simulink model "TruckBenchmark"  (R2023a)
settings: Solver=FixedStepAuto  StartTime=0.0  StopTime=sim_time  FixedStep=control.Ts  MaxStep=1  RelTol=1e-3  EnableMultiTasking=on
StartFcn:
  | tic
StopFcn:
  | simt=toc;
  | fprintf('Simulation time %.3f s\n',simt)
  | TruckBenchmark_Evaluation
values from neighbouring files (symbols this model uses):
  attack_duration = input('Enter the duration of each attack: ')    [RunMe.m]
  attack_freq = input('Enter the desired frequency of attack: ')    [RunMe.m]
  attack_time = input('Enter the time for attack: ')    [RunMe.m]
  attack_type = input('Select the type of Attack (1= Fuzzy, 2=spoofing, 3=Plateau, 4=Replay Attack, 5 = GAttack, 6= C-GAttack, 7= No Attack, 8 = Denial of Service):')    [RunMe.m]
  can_sample_time = 0.001    [runSim.m]
  clutch_pos = TruckBenchmark_Result.find('clutch_pos').Values    [TruckBenchmark_Evaluation.m]
  control =     [TruckBenchmark_Control.mat]
  cruise_profile = input('Select Cruise Profile (Step decrease = 1, Constant 80kph = 2): ')    [RunMe.m]
  curr_gear = TruckBenchmark_Result.find('curr_gear').Values    [TruckBenchmark_Evaluation.m]
  DoS = 0    [RunMe.m]
  gattack_data = interp1(original_time, data, desired_time, 'linear')    [RunMe.m]
  gattack_time = desired_time    [RunMe.m]
  k_slope = TruckBenchmark_Result.find('k_slope').Values    [TruckBenchmark_Evaluation.m]
  lambda = TruckBenchmark_Result.find('lambda').Values    [TruckBenchmark_Evaluation.m]
  model =     [TruckBenchmark_Data.mat]
  n_engine = TruckBenchmark_Result.find('n_engine').Values    [TruckBenchmark_Evaluation.m]
  road = scenario.road    [runSim.m]
  scenario =     [Sodertalje_Norrkoping_Scenario.mat]
  sim_time = input('Enter the total simulation time: ')    [RunMe.m]
  spoofed_value = input('Set the spoofing value:')    [RunMe.m]
  ts = struct('orig_30kph', ts_orig_30kph, 'gen_30kph', ts_gen_30kph, 'orig_40kph', ts_orig_40kph, 'gen_40kph', ts_gen_40kph, 'orig_50kph', ts_orig_50kph, 'gen_50kph', ts_gen_50kph, 'orig_60kph', ts_orig_60kph, 'gen_60kph', ts_gen_60kph,'orig_70kph', ts_orig_70kph, 'gen_70kph', ts_gen_70kph, 'orig_80kph', ts_orig_80kph, 'gen_80kph', ts_gen_80kph, 'orig_90kph', ts_orig_90kph, 'gen_90kph', ts_gen_90kph)    [data_to_mat.m]
  v_vehicle = 0    [RunMe.m]    (also in TruckBenchmark_Evaluation.m = TruckBenchmark_Result.find('v_vehicle').Values)
undefined symbols (not defined in the file or in its folder): canChannel, CCVS, DiscIntNeverNeededParam, dm_airInlet, EGF1, ESSI, ETC2, gcbh, IMT1, n_t, p_inletManifold, r_egr, VD, VDHR, x_distance
libraries: j1939protocollib x25, simulink x5, canlib x2, j1939tllib x2, canmsglib x1, vntj1939tllib x1, slpidlib x1
(part 1 of 4)
settings Model: PacingRate=100  Creator=SSSLRW  LastModifiedBy=kazishb
settings SolverCC: NumberNewtonIterations=2  SolverJacobianMethodControl=SparsePerturbation  AlgebraicLoopSolver=TrustRegion  AutoInsertRateTranBlk=on  InsertRTBMode=Never (minimum delay)
settings DataIOCC: LimitDataPoints=on  SaveFormat=Array  ReturnWorkspaceOutputs=off  SignalLoggingName=TruckBenchmark_Result
settings OptimizationCC: LifeSpan=inf
settings DebuggingCC: SolverPrmCheckMsg=warning  InheritedTsInSrcMsg=none  UnconnectedInputMsg=warning  UnconnectedOutputMsg=warning  UnconnectedLineMsg=warning  StrictBusMsg=ErrorOnBusTreatedAsVector  SFUnexpectedBacktrackingDiag=warning  SFNoUnconditionalDefaultTransitionDiag=warning  SFExecutionAtInitializationDiag=none  ArithmeticOperatorsInVariantConditions=warning
settings HardwareCC: ProdBitPerPointer=32  ProdBitPerSizeT=32  ProdBitPerPtrDiffT=32  ProdLargestAtomicFloat=None  ProdIntDivRoundTo=Undefined  ProdEndianess=Unspecified  ProdWordSize=32  ProdHWDeviceType=32-bit Generic
settings ModelReferenceCC: EnableRefExpFcnMdlSchedulingChecks=on  PropagateSignalLabelsOutOfModel=off
settings SFSimCC: SimUseLocalCustomCode=off  SimParseCustomCode=off  CustomCodeUndefinedFunction=UseInterfaceOnly
settings RTWCC: RTWUseLocalCustomCode=off
settings CodeAppCC: StateflowObjectComments=on
settings GRTTargetCC: TargetLangStandard=C89/C90 (ANSI)
settings ConfigComp: CovMetricSettings=dw  CovSaveCumulativeToWorkspaceVar=on  CovSaveSingleToWorkspaceVar=on  CovExternalEMLEnable=off

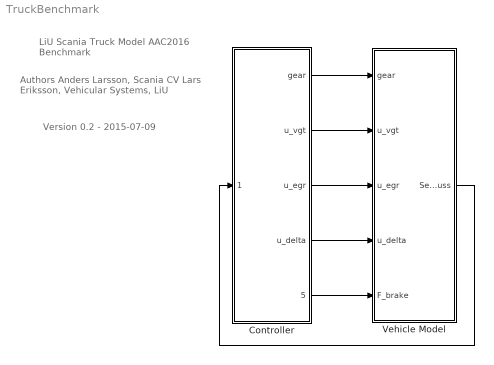
== system TruckBenchmark ==
  note: Version 0.2 - 2015-07-09
  note: Authors
      | Anders Larsson, Scania CV
      | Lars Eriksson, Vehicular Systems, LiU
  note: LiU Scania Truck Model
      | AAC2016 Benchmark
  Controller : Subsystem
  Vehicle Model : Subsystem
      settings: MinAlgLoopOccurrences=on
  wires:
  Vehicle Model/1(Sensor Buss) -> Controller/1(Sensors)
  Controller/1(gear) -> Vehicle Model/1(gear)
  Controller/2(u_vgt) -> Vehicle Model/2(u_vgt)
  Controller/3(u_egr) -> Vehicle Model/3(u_egr)
  Controller/4(u_delta) -> Vehicle Model/4(u_delta)
  Controller/5(u_brake) -> Vehicle Model/5(F_brake)

== system TruckBenchmark/Controller ==
  Sensors : Inport
  Bus Creator : BusCreator  Inputs=v_vehicle,clutch_pos,p_inletManifold,x_distance,dm_airInlet,n_engine,curr_gear,n_t,r_egr,lambda,k_slope
  Bus Selector : BusSelector  OutputSignals=v_vehicle,clutch_pos,x_distance,p_inletManifold,dm_airInlet,n_engine,curr_gear,n_t,r_egr,lambda,k_slope
  CAN TX/RX : Subsystem
  Controller : Subsystem  TreatAsAtomicUnit=on  SystemSampleTime=0.1
      settings: MinAlgLoopOccurrences=on
  Function-Call Generator : simulink/Ports & Subsystems/Function-Call Generator  sample_time=control.Ts  numberOfIterations=1  DisallowWideOutput=off
  Scope : Scope
  Scope1 : Scope
  Terminator1 : Terminator
  gear : Outport
  u_vgt : Outport  Port=2
  u_egr : Outport  Port=3
  u_delta : Outport  Port=4
  u_brake : Outport  Port=5
  wires:
  Controller/2(u_vgt) -> u_vgt/1
  Controller/1(gear) -> gear/1
  Controller/4(u_delta) -> u_delta/1
  Function-Call Generator/1 -> Controller/Trigger
  Controller/3(u_egr) -> u_egr/1
  Controller/5(F_brake) -> u_brake/1
  Bus Selector/2 -> CAN TX/RX/1(clutch_pos)  "<clutch_pos>"
  Bus Selector/3 -> CAN TX/RX/2(Vehicle Distance)  "<x_distance>"
  Bus Selector/4 -> Bus Creator/3, CAN TX/RX/3(Inlet Manifold Pressure)  "<p_inletManifold>"
  Bus Selector/5 -> CAN TX/RX/4(Compressor Air Mass Flow)  "<dm_airInlet>"
  Bus Selector/6 -> CAN TX/RX/5(Engine Speed)  "<n_engine>"
  Bus Selector/7 -> CAN TX/RX/6(Current Gear)  "<curr_gear>"
  Bus Selector/1 -> Scope/1, CAN TX/RX/7(v_vehicle)  "<v_vehicle>"
  CAN TX/RX/4(rx trip distance) -> Bus Creator/4  "x_distance"
  CAN TX/RX/5(rx Compressor Air Mass Flow) -> Bus Creator/5  "dm_airInlet"
  Bus Selector/8 -> CAN TX/RX/8(n_t_in)  "<n_t>"
  Bus Selector/9 -> CAN TX/RX/9(r_egr_in)  "<r_egr>"
  Bus Selector/10 -> CAN TX/RX/10(lambda_in)  "<lambda>"
  Bus Selector/11 -> CAN TX/RX/11(k_slope_in)  "<k_slope>"
  CAN TX/RX/8(n_t) -> Bus Creator/8
  CAN TX/RX/9(r_egr) -> Bus Creator/9
  CAN TX/RX/10(lambda) -> Bus Creator/10
  CAN TX/RX/11(k_slope) -> Bus Creator/11
  CAN TX/RX/1(rx Vehicle Velocity) -> Scope1/1, Bus Creator/1  "v_vehicle"
  CAN TX/RX/2(rx Clutch Position) -> Bus Creator/2  "clutch_pos"
  CAN TX/RX/7(rx Current Gear) -> Bus Creator/7  "curr_gear"
  CAN TX/RX/6(rx Engine Speed) -> Bus Creator/6  "n_engine"
  Sensors/1 -> Bus Selector/1
  Bus Creator/1 -> Controller/1(Sensor Bus)
  CAN TX/RX/3(rx Inlet Manifold Pressure) -> Terminator1/1  "p_inletManifold"
  Controller/6(cruise_set_speed) -> CAN TX/RX/12(cruise_set_speed)

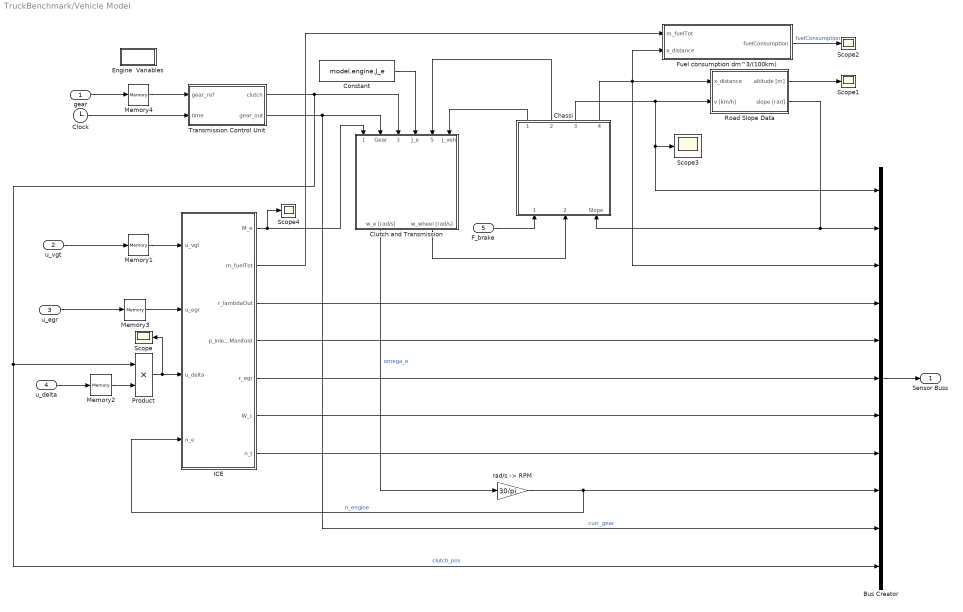
== system TruckBenchmark/Vehicle Model ==
  gear : Inport
  u_vgt : Inport  Port=2
  u_egr : Inport  Port=3
  u_delta : Inport  Port=4
  F_brake : Inport  Port=5
  Bus Creator : BusCreator  Inputs=11
  Chassi : Subsystem
  Clock : Clock
  Clutch and Transmission : Subsystem
  Constant : Constant  Value=model.engine.J_e
  Engine  Variables : Subsystem
  Fuel consumption dm^3/(100km) : MATLAB Function  TreatAsAtomicUnit=on
  ICE : Subsystem  mask{gamma_e=model.engine.gamma_e, gamma_a=model.engine.gamma_a, p_amb=model.engine.p_amb, c_ve=model.engine.c_ve, c_va=model.engine.c_va, c_pe=model.engine.c_pe, c_pa=model.engine.c_pa, T_im=model.engine.T_im, T_amb=model.engine.T_amb, R_e=model.engine.R_e, R_a=model.engine.R_a, X_Oc=model.engine.X_Oc, limit_m_f=model.engine.limit_m_f, limit_n_e=model.engine.limit_n_e}
      mask prompts: limit_m_f "m_f_limit"; limit_n_e "n_e_limit"
      mask help:
      | A model for a Diesel engine with EGT and VGT.
      |
      | The model is develped and parameterized for a Scania heavy duty truck engine and documented in the paper:
      |
      | Johan Wahlstrom and Lars Eriksson.
      | Modeling diesel engines with a variable-geometry turbocharger and exhaust gas recirculation by optimization of model parameters for capturing non-linear system dynamics.
      | Proceedings of the Institution of Mechanical Engineers, Part D, Journal of Automobile Engineering, Volume 225, Issue 7, July 2011.
      | http://dx.doi.org/10.1177/0954407011398177
      mask Help: To see the details of the model right click on the model select "Look Under Mask".
  Memory1 : Memory  InitialCondition=40
  Memory2 : Memory
  Memory3 : Memory
  Memory4 : Memory  InitialCondition=scenario.gear_init
  "Product " : Product  Inputs=**
  Road Slope Data : Subsystem
  Scope{,1..4} (5 alike) : Scope
  Transmission Control Unit : MATLAB Function  TreatAsAtomicUnit=on
  "rad/s -> RPM" : Gain  Gain=30/pi  SaturateOnIntegerOverflow=on  OutDataTypeStr=Inherit: Same as input  ParamDataTypeStr=Inherit: Same as input
  Sensor Buss : Outport  VectorParamsAs1DForOutWhenUnconnected=off
  wires:
  ICE/1(M_e) -> Clutch and Transmission/1(M_e [Nm]), Scope4/1
  Road Slope Data/2(slope [rad]) -> Chassi/3(Slope), Bus Creator/2
  Chassi/3(Vehicle Speed[km/h]) -> Road Slope Data/2(v [km/h]), Bus Creator/1, Scope3/1
  ICE/2(m_fuelTot) -> Fuel consumption dm^3/(100km)/1(m_fuelTot)
  Fuel consumption dm^3/(100km)/1(fuelConsumption) -> Scope2/1  "fuelConsumption"
  Chassi/4(Distance [m]) -> Road Slope Data/1(x_distance), Fuel consumption dm^3/(100km)/2(x_distance), Bus Creator/3
  ICE/3(r_lambdaOut) -> Bus Creator/4
  ICE/4(p_inletManifold) -> Bus Creator/5
  ICE/5(r_egr) -> Bus Creator/6
  ICE/6(W_c) -> Bus Creator/7
  u_vgt/1 -> Memory1/1
  u_egr/1 -> Memory3/1
  Memory3/1 -> ICE/2(u_egr)
  F_brake/1 -> Chassi/1(Brake Pedal [%])
  Bus Creator/1 -> Sensor Buss/1
  Clutch and Transmission/2(w_wheel [rad/s]) -> Chassi/2(Wheel speed [rad/s])
  Clutch and Transmission/1(w_e [rad/s]) -> "rad/s -> RPM"/1  "omega_e"
  Chassi/1(Vehicle Inertia [kgm^2]) -> Clutch and Transmission/6(J_veh)
  Chassi/2(Vehicle Torque [Nm]) -> Clutch and Transmission/5(M_veh [Nm])
  "rad/s -> RPM"/1 -> ICE/4(n_e), Bus Creator/9  "n_engine"
  Constant/1 -> Clutch and Transmission/4(J_e)
  Memory1/1 -> ICE/1(u_vgt)
  Transmission Control Unit/2(gear_out) -> Bus Creator/10, Clutch and Transmission/2(Gear)  "curr_gear"
  Clock/1 -> Transmission Control Unit/2(time)
  gear/1 -> Memory4/1
  "Product "/1 -> Scope/1, ICE/3(u_delta)
  Transmission Control Unit/1(clutch) -> Clutch and Transmission/3(Clutch Pos [0...1]), "Product "/1, Bus Creator/11  "clutch_pos"
  u_delta/1 -> Memory2/1
  Memory4/1 -> Transmission Control Unit/1(gear_ref)
  ICE/7(n_t) -> Bus Creator/8
  Road Slope Data/1(altitude [m]) -> Scope1/1
  Memory2/1 -> "Product "/2

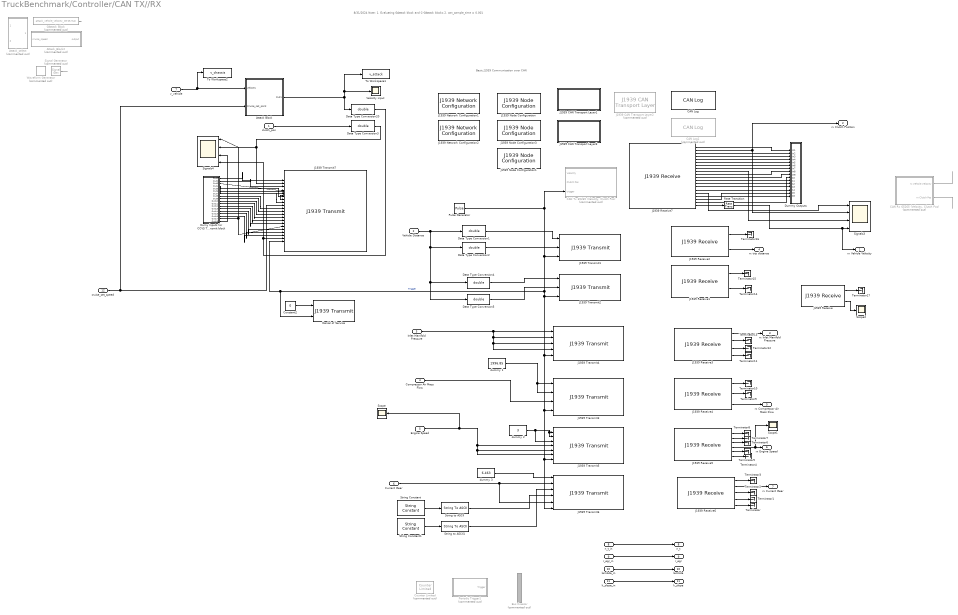
== system TruckBenchmark/Controller/CAN TX//RX ==
  note: 8/31/2024
      | Note:
      | 1. Evaluating GAttack block and C-GAttack blocks
      | 2. can_sample_time = 0.001
  note: Basic J1939 Communication over CAN
  clutch_pos : Inport
  Vehicle Distance : Inport  Port=2
  Inlet Manifold Pressure : Inport  Port=3
  Compressor Air Mass Flow : Inport  Port=4
  Engine Speed : Inport  Port=5
  Current Gear : Inport  Port=6
  v_vehicle : Inport  Port=7
  n_t_in : Inport  Port=8
  r_egr_in : Inport  Port=9
  lambda_in : Inport  Port=10
  k_slope_in : Inport  Port=11
  cruise_set_speed : Inport  Port=12
  " Periodic Trigger1" : Subsystem  Commented=on  mask(PeriodicTrigger){repetitionInterval=1}
      mask prompts: repetitionInterval "Repetition Interval (ms):"
      mask help: This block uses the wall-clock time to periodically output a trigger pulse
      mask init:
      | if repetitionInterval < 0
      |  error('xPCTarget:xpcblocks:j1939messagetrigger',...
      |        'Repetition Interval cannot be less than zero');
      | end
      mask Display: disp('Periodic Trigger \n Subsystem');
  Attack Block : Subsystem
  Attack_Block2 : MATLAB Function  Commented=on  TreatAsAtomicUnit=on
  Attack_select : MATLAB Function  Commented=on  TreatAsAtomicUnit=on
  Bus Creator : BusCreator  Commented=on  Inputs=2
  CAN Log : canlib/CAN Log  BlockHandle=376.0004  FullPathFileName=can_raw_virtual.mat  FileName=can_raw_virtual.mat  VariableName=CAN_BUS_virtual  MaxNumMessages=100000000  LogFrom=CAN Bus  DeviceMenu=MathWorks Virtual 1 (Channel 2)  Device=MathWorks Virtual 1 (Channel 2)  ObjConstructor=canChannel('MathWorks', 'Virtual 1', 2)  SampleTime=can_sample_time
  CAN Log1 : canlib/CAN Log  Commented=on  BlockHandle=377.0001  FullPathFileName=can_raw_pcan.mat  FileName=can_raw_pcan.mat  VariableName=CAN_BUS_pcan  MaxNumMessages=100000000  LogFrom=CAN Bus  DeviceMenu=Select a device  Device=PEAK-System PCAN-USB (PCAN_USBBUS1)  ObjConstructor=canChannel('MathWorks', 'Virtual 1', 2)  SampleTime=can_sample_time
  "CAN Rx 65265 (Velocity, Clutch Pos)" : Subsystem  Commented=on
  "CAN Tx 65265 (Velocity, Clutch Pos)" : Subsystem  Commented=on
  Constant2 : Constant  Value=0
  Counter Limited : simulink/Sources/Counter Limited  Commented=on  uplimit=7  tsamp=0.1
  Data Type Conversion{1..5,20} (6 alike) : DataTypeConversion  OutDataTypeStr=double  SaturateOnIntegerOverflow=off  RndMeth=Floor
  Denial of Service : j1939protocollib/J1939 Transmit  Priority=-1  ConfigName=Config2  NodeName=Engine1  PGList=DoS(0)  PGName=DoS  MsgLength=8  SignalInfo=DenialofService$0$16$1$2$1$0$2.500000e-03$0$0$1.606375e+02$%$0$#  NSignals=1  StartBits=str2num('[double(0)]')  SignalSizes=str2num('[double(16)]')  ByteOrders=str2num('[int32(1)]')  DataTypes=str2num('[int32(2)]')  MultiplexTypes=str2num('[int32(1)]')  MultiplexValues=str2num('[double(0)]')  Factors=str2num('[double(2.500000e-03)]')  Offsets=str2num('[double(0)]')  Minimums=str2num('[double(0)]')  Maximums=str2num('[double(1.606375e+02)]')  Units=0  SPN=str2num('[double(0)]')  Comment=0  PGPriority=0  DestAddrID=Custom  DestAddrName=255  TransmitPeriodically=on  MessagePeriod=0  SampleTime=-1  ApplyMinMax=off
      settings: LibrarySourceBlock=vntj1939lib/J1939 Transmit
  Dummy Outputs : Subsystem
  Dumy Inputs for CCVS Transmit block : Subsystem
  GAttack Block : FromFile  Commented=on  FileName=attack_vehicle_velocity_03-25.mat  OutDataTypeStr=double  SampleTime=can_sample_time
  J1939 CAN Transport Layer1 : Subsystem  Priority=-2  AncestorBlock=vntj1939tllib/J1939 CAN Transport Layer  DialogController=vntcreatedialog  TreatAsAtomicUnit=on  mask(J1939 CAN Transport Layer){DeviceMenu=MathWorks Virtual 1 (Channel 1), ConfigName=Config1, ObjConstructor=canChannel('MathWorks', 'Virtual 1', 1), Device=MathWorks Virtual 1 (Channel 1), BusSpeedStr=250000, SampleTime=can_sample_time}
      mask prompts: DeviceMenu "Device:"; ConfigName "Config name:"; ObjConstructor "Object Constructor"; Device "Device Name"; BusSpeedStr "Bus speed"; SampleTime "Sample time"
      mask help:
      | Handles receiving and transmitting J1939 messages over CAN
      | using the specified device.
      mask init:
      | dispString = j1939sl.internal.getDisplayString;
      settings: LibrarySourceBlock=|
      | vntj1939tllib/J1939 CAN
      | Transport Layer
      mask Help: helpview('vnt', 'vnt_j1939_can_tl');
      mask TypeOptions DeviceMenu: Select a device | MathWorks Virtual 1 (Channel 1) | MathWorks Virtual 1 (Channel 2) | (none)
      mask Display: disp(dispString);
  J1939 CAN Transport Layer2 : vntj1939tllib/J1939 CAN Transport Layer  Priority=-2  Commented=on  DeviceMenu=Select a device  ConfigName=Config2  ObjConstructor=canChannel('PEAK-System', 'PCAN_USBBUS1')  Device=PEAK-System PCAN-USB (PCAN_USBBUS1)  BusSpeedStr=250000  SampleTime=can_sample_time
      settings: LibrarySourceBlock=|
      | vntj1939lib/J1939 CAN
      | Transport Layer
  J1939 CAN Transport Layer3 : Subsystem  Priority=-2  AncestorBlock=vntj1939tllib/J1939 CAN Transport Layer  DialogController=vntcreatedialog  TreatAsAtomicUnit=on  mask(J1939 CAN Transport Layer){DeviceMenu=MathWorks Virtual 1 (Channel 2), ConfigName=Config2, ObjConstructor=canChannel('MathWorks', 'Virtual 1', 2), Device=MathWorks Virtual 1 (Channel 2), BusSpeedStr=250000, SampleTime=can_sample_time}
      mask prompts: DeviceMenu "Device:"; ConfigName "Config name:"; ObjConstructor "Object Constructor"; Device "Device Name"; BusSpeedStr "Bus speed"; SampleTime "Sample time"
      mask help:
      | Handles receiving and transmitting J1939 messages over CAN
      | using the specified device.
      mask init:
      | dispString = j1939sl.internal.getDisplayString;
      settings: LibrarySourceBlock=|
      | vntj1939tllib/J1939 CAN
      | Transport Layer
      mask Help: helpview('vnt', 'vnt_j1939_can_tl');
      mask TypeOptions DeviceMenu: Select a device | MathWorks Virtual 1 (Channel 1) | MathWorks Virtual 1 (Channel 2) | (none)
      mask Display: disp(dispString);
  J1939 Network Configuration1 : j1939protocollib/J1939 Network Configuration  Priority=-3  ConfigName=Config1  DbFile=C:\Users\qazim\OneDrive - The Ohio State University\Application for Fellowship\.Project\SDCS\J1939 Standards\j1939.dbc  PrevDbFile=C:\Users\qazim\OneDrive - The Ohio State University\Application for Fellowship\.Project\SDCS\J1939 Standards\j1939.dbc
  J1939 Network Configuration2 : j1939protocollib/J1939 Network Configuration  Priority=-3  ConfigName=Config2  DbFile=C:\Users\qazim\OneDrive - The Ohio State University\Application for Fellowship\.Project\SDCS\Papers\!Research Paper\SAE WCX 2024\j1939.dbc  PrevDbFile=C:\Users\qazim\OneDrive - The Ohio State University\Application for Fellowship\.Project\SDCS\Papers\!Research Paper\SAE WCX 2024\j1939.dbc
  J1939 Node Configuration : j1939protocollib/J1939 Node Configuration  Priority=-2  ConfigName=Config1  NodeID=Engine1  NodeName=Engine1  PrevNodeID=Custom  PrevConfig=Config  AllowAAC=off  NodeAddress=0  IndustryGroup=0  VehicleSystem=0  VehicleSystemInstance=0  FunctionID=0  FunctionInstance=0  ECUInstance=0  ManufacturerCode=0  IDNumber=0  SampleTime=-1  OutputAddress=off  OutputACStatus=off
  J1939 Node Configuration1 : j1939protocollib/J1939 Node Configuration  Priority=-2  ConfigName=Config2  NodeID=Transmission1  NodeName=Transmission1  PrevNodeID=Custom  PrevConfig=Config  AllowAAC=off  NodeAddress=3  IndustryGroup=0  VehicleSystem=0  VehicleSystemInstance=0  FunctionID=3  FunctionInstance=0  ECUInstance=0  ManufacturerCode=0  IDNumber=0  SampleTime=can_sample_time  OutputAddress=off  OutputACStatus=off
  J1939 Node Configuration3 : j1939protocollib/J1939 Node Configuration  Priority=-2  ConfigName=Config2  NodeID=Engine1  NodeName=Engine1  PrevNodeID=Custom  PrevConfig=Config  AllowAAC=off  NodeAddress=0  IndustryGroup=0  VehicleSystem=0  VehicleSystemInstance=0  FunctionID=0  FunctionInstance=0  ECUInstance=0  ManufacturerCode=0  IDNumber=0  SampleTime=can_sample_time  OutputAddress=off  OutputACStatus=off
  J1939 Receive : j1939protocollib/J1939 Receive  Priority=-1  ConfigName=Config2  NodeName=Engine1  PGList=DoS(0)  PGName=DoS  MsgLength=8  SignalInfo=DenialofService$0$16$1$2$1$0$2.500000e-03$0$0$1.606375e+02$%$0$#  NSignals=1  StartBits=str2num('[double(0)]')  SignalSizes=str2num('[double(16)]')  ByteOrders=str2num('[int32(1)]')  DataTypes=str2num('[int32(2)]')  MultiplexTypes=str2num('[int32(1)]')  MultiplexValues=str2num('[double(0)]')  Factors=str2num('[double(2.500000e-03)]')  Offsets=str2num('[double(0)]')  Minimums=str2num('[double(0)]')  Maximums=str2num('[double(1.606375e+02)]')  Units=0  SPN=str2num('[double(0)]')  Comment=0  SrcAddrFilter=Allow all  SrcAddress=255  DestAddrFilter=1  outputNew=on  SampleTime=0.01  ApplyMinMax=off
      settings: LibrarySourceBlock=vntj1939lib/J1939 Receive
  J1939 Receive1 : j1939protocollib/J1939 Receive  Priority=-1  ConfigName=Config2  NodeName=Engine1  PGList=VD(65248)  PGName=VD  MsgLength=8  SignalInfo=TotalVehicleDistance$32$32$1$2$1$0$1.250000e-01$0$0$5.263852e+08$km$245$#TripDistance$0$32$1$2$1$0$1.250000e-01$0$0$5.263852e+08$km$244$#  NSignals=2  StartBits=str2num('[double(32);double(0)]')  SignalSizes=str2num('[double(32),double(32)]')  ByteOrders=str2num('[int32(1);int32(1)]')  DataTypes=str2num('[int32(2);int32(2)]')  MultiplexTypes=str2num('[int32(1);int32(1)]')  MultiplexValues=str2num('[double(0);double(0)]')  Factors=str2num('[double(1.250000e-01);double(1.250000e-01)]')  Offsets=str2num('[double(0);double(0)]')  Minimums=str2num('[double(0);double(0)]')  Maximums=str2num('[double(5.263852e+08);double(5.263852e+08)]')  Units=0  SPN=str2num('[double(245);double(244)]')  Comment=0  SrcAddrFilter=Allow all  SrcAddress=255  DestAddrFilter=1  outputNew=off  SampleTime=can_sample_time  ApplyMinMax=off
  J1939 Receive2 : j1939protocollib/J1939 Receive  Priority=-1  ConfigName=Config2  NodeName=Engine1  PGList=VDHR(65217)  PGName=VDHR  MsgLength=8  SignalInfo=HghRslutionTotalVehicleDistance$0$32$1$2$1$0$5$0$0$21055406$km$917$#HighResolutionTripDistance$32$32$1$2$1$0$5$0$0$21055406$km$918$#  NSignals=2  StartBits=str2num('[double(0);double(32)]')  SignalSizes=str2num('[double(32),double(32)]')  ByteOrders=str2num('[int32(1);int32(1)]')  DataTypes=str2num('[int32(2);int32(2)]')  MultiplexTypes=str2num('[int32(1);int32(1)]')  MultiplexValues=str2num('[double(0);double(0)]')  Factors=str2num('[double(5);double(5)]')  Offsets=str2num('[double(0);double(0)]')  Minimums=str2num('[double(0);double(0)]')  Maximums=str2num('[double(21055406);double(21055406)]')  Units=0  SPN=str2num('[double(917);double(918)]')  Comment=0  SrcAddrFilter=Allow all  SrcAddress=255  DestAddrFilter=2  outputNew=off  SampleTime=can_sample_time  ApplyMinMax=off
  J1939 Receive3 : j1939protocollib/J1939 Receive  Priority=-1  ConfigName=Config2  NodeName=Engine1  PGList=IMT1(65190)  PGName=IMT1  MsgLength=8  SignalInfo=EngTurbo1BoostPress$0$16$1$2$1$0$1.250000e-01$0$0$8.031875e+03$kPa$1127$#EngTurbo2BoostPress$16$16$1$2$1$0$1.250000e-01$0$0$8.031875e+03$kPa$1128$#EngTurbo3BoostPress$32$16$1$2$1$0$1.250000e-01$0$0$8.031875e+03$kPa$1129$#EngTurbo4BoostPress$48$16$1$2$1$0$1.250000e-01$0$0$8.031875e+03$kPa$1130$#  NSignals=4  StartBits=str2num('[double(0);double(16);double(32);double(48)]')  SignalSizes=str2num('[double(16),double(16),double(16),double(16)]')  ByteOrders=str2num('[int32(1);int32(1);int32(1);int32(1)]')  DataTypes=str2num('[int32(2);int32(2);int32(2);int32(2)]')  MultiplexTypes=str2num('[int32(1);int32(1);int32(1);int32(1)]')  MultiplexValues=str2num('[double(0);double(0);double(0);double(0)]')  Factors=str2num('[double(1.250000e-01);double(1.250000e-01);double(1.250000e-01);double(1.250000e-01)]')  Offsets=str2num('[double(0);double(0);double(0);double(0)]')  Minimums=str2num('[double(0);double(0);double(0);double(0)]')  Maximums=str2num('[double(8.031875e+03);double(8.031875e+03);double(8.031875e+03);double(8.031875e+03)]')  Units=0  SPN=str2num('[double(1127);double(1128);double(1129);double(1130)]')  Comment=0  SrcAddrFilter=Allow all  SrcAddress=255  DestAddrFilter=2  outputNew=off  SampleTime=can_sample_time  ApplyMinMax=off
  J1939 Receive4 : j1939protocollib/J1939 Receive  Priority=-1  ConfigName=Config2  NodeName=Engine1  PGList=EGF1(61450)  PGName=EGF1  MsgLength=8  SignalInfo=EngExhstGsRcrclton1MassFlowRate$0$16$1$2$1$0$5.000000e-02$0$0$3.212750e+03$kg/h$2659$#EngExhstGsRcrclton2MassFlowRate$32$16$1$2$1$0$5.000000e-02$0$0$3.212750e+03$kg/h$5257$#EngIntakeAirMassFlowRate$16$16$1$2$1$0$5.000000e-02$0$0$3.212750e+03$kg/h$132$#  NSignals=3  StartBits=str2num('[double(0);double(32);double(16)]')  SignalSizes=str2num('[double(16),double(16),double(16)]')  ByteOrders=str2num('[int32(1);int32(1);int32(1)]')  DataTypes=str2num('[int32(2);int32(2);int32(2)]')  MultiplexTypes=str2num('[int32(1);int32(1);int32(1)]')  MultiplexValues=str2num('[double(0);double(0);double(0)]')  Factors=str2num('[double(5.000000e-02);double(5.000000e-02);double(5.000000e-02)]')  Offsets=str2num('[double(0);double(0);double(0)]')  Minimums=str2num('[double(0);double(0);double(0)]')  Maximums=str2num('[double(3.212750e+03);double(3.212750e+03);double(3.212750e+03)]')  Units=0  SPN=str2num('[double(2659);double(5257);double(132)]')  Comment=0  SrcAddrFilter=Allow all  SrcAddress=255  DestAddrFilter=2  outputNew=off  SampleTime=can_sample_time  ApplyMinMax=off
  J1939 Receive5 : j1939protocollib/J1939 Receive  Priority=-1  ConfigName=Config2  NodeName=Engine1  PGList=ESSI(61473)  PGName=ESSI  MsgLength=8  SignalInfo=EngSpdSnsor1TimingPatternStatus$54$2$1$2$1$0$1$0$0$3$$4203$#EngSpdSnsor2TimingPatternStatus$52$2$1$2$1$0$1$0$0$3$$4204$#EngSpdSnsor3TimingPatternStatus$50$2$1$2$1$0$1$0$0$3$$4205$#EngSpeed1$0$16$1$2$1$0$5.000000e-01$0$0$3.212750e+04$rpm$4201$#EngSpeed2$16$16$1$2$1$0$5.000000e-01$0$0$3.212750e+04$rpm$723$#EngSpeed3$32$16$1$2$1$0$5.000000e-01$0$0$3.212750e+04$rpm$4202$#  NSignals=6  StartBits=str2num('[double(54);double(52);double(50);double(0);double(16);double(32)]')  SignalSizes=str2num('[double(2),double(2),double(2),double(16),double(16),double(16)]')  ByteOrders=str2num('[int32(1);int32(1);int32(1);int32(1);int32(1);int32(1)]')  DataTypes=str2num('[int32(2);int32(2);int32(2);int32(2);int32(2);int32(2)]')  MultiplexTypes=str2num('[int32(1);int32(1);int32(1);int32(1);int32(1);int32(1)]')  MultiplexValues=str2num('[double(0);double(0);double(0);double(0);double(0);double(0)]')  Factors=str2num('[double(1);double(1);double(1);double(5.000000e-01);double(5.000000e-01);double(5.000000e-01)]')  Offsets=str2num('[double(0);double(0);double(0);double(0);double(0);double(0)]')  Minimums=str2num('[double(0);double(0);double(0);double(0);double(0);double(0)]')  Maximums=str2num('[double(3);double(3);double(3);double(3.212750e+04);double(3.212750e+04);double(3.212750e+04)]')  Units=0  SPN=str2num('[double(4203);double(4204);double(4205);double(4201);double(723);double(4202)]')  Comment=0  SrcAddrFilter=Allow all  SrcAddress=255  DestAddrFilter=2  outputNew=off  SampleTime=can_sample_time  ApplyMinMax=off
  J1939 Receive6 : j1939protocollib/J1939 Receive  Priority=-1  ConfigName=Config2  NodeName=Transmission1  PGList=ETC2(61445)  PGName=ETC2  MsgLength=8  SignalInfo=TransActualGearRatio$8$16$1$2$1$0$1.000000e-03$0$0$6.425500e+01$$526$#TransCurrentGear$24$8$1$2$1$0$1$-125$-125$125$$523$#TransCurrentRange$48$16$1$2$1$0$1$0$0$255$$163$#TransRqedRange$32$16$1$2$1$0$1$0$0$255$per$162$#TransSelectedGear$0$8$1$2$1$0$1$-125$-125$125$$524$#  NSignals=5  StartBits=str2num('[double(8);double(24);double(48);double(32);double(0)]')  SignalSizes=str2num('[double(16),double(8),double(16),double(16),double(8)]')  ByteOrders=str2num('[int32(1);int32(1);int32(1);int32(1);int32(1)]')  DataTypes=str2num('[int32(2);int32(2);int32(2);int32(2);int32(2)]')  MultiplexTypes=str2num('[int32(1);int32(1);int32(1);int32(1);int32(1)]')  MultiplexValues=str2num('[double(0);double(0);double(0);double(0);double(0)]')  Factors=str2num('[double(1.000000e-03);double(1);double(1);double(1);double(1)]')  Offsets=str2num('[double(0);double(-125);double(0);double(0);double(-125)]')  Minimums=str2num('[double(0);double(-125);double(0);double(0);double(-125)]')  Maximums=str2num('[double(6.425500e+01);double(125);double(255);double(255);double(125)]')  Units=0  SPN=str2num('[double(526);double(523);double(163);double(162);double(524)]')  Comment=0  SrcAddrFilter=Allow all  SrcAddress=255  DestAddrFilter=2  outputNew=off  SampleTime=can_sample_time  ApplyMinMax=off
  J1939 Receive7 : j1939protocollib/J1939 Receive  Priority=-1  ConfigName=Config2  NodeName=Engine1  PGList=CCVS(65265)  PGName=CCVS  MsgLength=8  SignalInfo=BrakeSwitch$28$2$1$2$1$0$1$0$0$3$$597$#ClutchSwitch$30$2$1$2$1$0$1$0$0$3$$598$#CruiseCtrlAccelerateSwitch$38$2$1$2$1$0$1$0$0$3$$602$#CruiseCtrlActive$24$2$1$2$1$0$1$0$0$3$$595$#CruiseCtrlCoastSwitch$34$2$1$2$1$0$1$0$0$3$$600$#CruiseCtrlEnableSwitch$26$2$1$2$1$0$1$0$0$3$$596$#CruiseCtrlPauseSwitch$4$2$1$2$1$0$1$0$0$3$$1633$#CruiseCtrlResumeSwitch$36$2$1$2$1$0$1$0$0$3$$601$#CruiseCtrlSetSpeed$40$8$1$2$1$0$1$0$0$250$km/h$86$#CruiseCtrlSetSwitch$32$2$1$2$1$0$1$0$0$3$$599$#CruiseCtrlStates$53$3$1$2$1$0$1$0$0$7$$527$#EngIdleDecrementSwitch$58$2$1$2$1$0$1$0$0$3$$967$#EngIdleIncrementSwitch$56$2$1$2$1$0$1$0$0$3$$968$#EngShutdownOverrideSwitch$62$2$1$2$1$0$1$0$0$3$$1237$#EngTestModeSwitch$60$2$1$2$1$0$1$0$0$3$$966$#PTOGovernorState$48$5$1$2$1$0$1$0$0$31$$976$#ParkBrakeReleaseInhibitRq$6$2$1$2$1$0$1$0$0$3$$3807$#ParkingBrakeSwitch$2$2$1$2$1$0$1$0$0$3$$70$#TwoSpeedAxleSwitch$0$2$1$2$1$0$1$0$0$3$$69$#WheelBasedVehicleSpeed$8$16$1$2$1$0$3.906250e-03$0$0$2.509960e+02$km/h$84$#  NSignals=20  StartBits=str2num('[double(28);double(30);double(38);double(24);double(34);double(26);double(4);double(36);double(40);double(32);double(53);double(58);double(56);double(62);double(60);double(48);double(6);double(2);double(0);double(8)]')  SignalSizes=str2num('[double(2),double(2),double(2),double(2),double(2),double(2),double(2),double(2),double(8),double(2),double(3),double(2),double(2),double(2),double(2),double(5),double(2),double(2),double(2),double(16)]')  ByteOrders=str2num('[int32(1);int32(1);int32(1);int32(1);int32(1);int32(1);int32(1);int32(1);int32(1);int32(1);int32(1);int32(1);int32(1);int32(1);int32(1);int32(1);int32(1);int32(1);int32(1);int32(1)]')  DataTypes=str2num('[int32(2);int32(2);int32(2);int32(2);int32(2);int32(2);int32(2);int32(2);int32(2);int32(2);int32(2);int32(2);int32(2);int32(2);int32(2);int32(2);int32(2);int32(2);int32(2);int32(2)]')  MultiplexTypes=str2num('[int32(1);int32(1);int32(1);int32(1);int32(1);int32(1);int32(1);int32(1);int32(1);int32(1);int32(1);int32(1);int32(1);int32(1);int32(1);int32(1);int32(1);int32(1);int32(1);int32(1)]')  MultiplexValues=str2num('[double(0);double(0);double(0);double(0);double(0);double(0);double(0);double(0);double(0);double(0);double(0);double(0);double(0);double(0);double(0);double(0);double(0);double(0);double(0);double(0)]')  Factors=str2num('[double(1);double(1);double(1);double(1);double(1);double(1);double(1);double(1);double(1);double(1);double(1);double(1);double(1);double(1);double(1);double(1);double(1);double(1);double(1);double(3.906250e-03)]')  Offsets=str2num('[double(0);double(0);double(0);double(0);double(0);double(0);double(0);double(0);double(0);double(0);double(0);double(0);double(0);double(0);double(0);double(0);double(0);double(0);double(0);double(0)]')  Minimums=str2num('[double(0);double(0);double(0);double(0);double(0);double(0);double(0);double(0);double(0);double(0);double(0);double(0);double(0);double(0);double(0);double(0);double(0);double(0);double(0);double(0)]')  Maximums=str2num('[double(3);double(3);double(3);double(3);double(3);double(3);double(3);double(3);double(250);double(3);double(7);double(3);double(3);double(3);double(3);double(31);double(3);double(3);double(3);double(2.509960e+02)]')  Units=0  SPN=str2num('[double(597);double(598);double(602);double(595);double(600);double(596);double(1633);double(601);double(86);double(599);double(527);double(967);double(968);double(1237);double(966);double(976);double(3807);double(70);double(69);double(84)]')  Comment=0  SrcAddrFilter=Allow all  SrcAddress=255  DestAddrFilter=2  outputNew=off  SampleTime=can_sample_time  ApplyMinMax=off
  J1939 Transmit1 : j1939protocollib/J1939 Transmit  Priority=-1  ConfigName=Config1  NodeName=Engine1  PGList=VDHR(65217)  PGName=VDHR  MsgLength=8  SignalInfo=HghRslutionTotalVehicleDistance$0$32$1$2$1$0$5$0$0$21055406$km$917$#HighResolutionTripDistance$32$32$1$2$1$0$5$0$0$21055406$km$918$#  NSignals=2  StartBits=str2num('[double(0);double(32)]')  SignalSizes=str2num('[double(32),double(32)]')  ByteOrders=str2num('[int32(1);int32(1)]')  DataTypes=str2num('[int32(2);int32(2)]')  MultiplexTypes=str2num('[int32(1);int32(1)]')  MultiplexValues=str2num('[double(0);double(0)]')  Factors=str2num('[double(5);double(5)]')  Offsets=str2num('[double(0);double(0)]')  Minimums=str2num('[double(0);double(0)]')  Maximums=str2num('[double(21055406);double(21055406)]')  Units=0  SPN=str2num('[double(917);double(918)]')  Comment=0  PGPriority=6  DestAddrID=Custom  DestAddrName=255  TransmitPeriodically=on  MessagePeriod=0  SampleTime=can_sample_time  ApplyMinMax=off
  J1939 Transmit2 : j1939protocollib/J1939 Transmit  Priority=-1  ConfigName=Config1  NodeName=Engine1  PGList=VD(65248)  PGName=VD  MsgLength=8  SignalInfo=TotalVehicleDistance$32$32$1$2$1$0$1.250000e-01$0$0$5.263852e+08$km$245$#TripDistance$0$32$1$2$1$0$1.250000e-01$0$0$5.263852e+08$km$244$#  NSignals=2  StartBits=str2num('[double(32);double(0)]')  SignalSizes=str2num('[double(32),double(32)]')  ByteOrders=str2num('[int32(1);int32(1)]')  DataTypes=str2num('[int32(2);int32(2)]')  MultiplexTypes=str2num('[int32(1);int32(1)]')  MultiplexValues=str2num('[double(0);double(0)]')  Factors=str2num('[double(1.250000e-01);double(1.250000e-01)]')  Offsets=str2num('[double(0);double(0)]')  Minimums=str2num('[double(0);double(0)]')  Maximums=str2num('[double(5.263852e+08);double(5.263852e+08)]')  Units=0  SPN=str2num('[double(245);double(244)]')  Comment=0  PGPriority=6  DestAddrID=Custom  DestAddrName=255  TransmitPeriodically=on  MessagePeriod=0  SampleTime=can_sample_time  ApplyMinMax=off
  J1939 Transmit3 : j1939protocollib/J1939 Transmit  Priority=-1  ConfigName=Config1  NodeName=Engine1  PGList=EGF1(61450)  PGName=EGF1  MsgLength=8  SignalInfo=EngExhstGsRcrclton1MassFlowRate$0$16$1$2$1$0$5.000000e-02$0$0$3.212750e+03$kg/h$2659$#EngExhstGsRcrclton2MassFlowRate$32$16$1$2$1$0$5.000000e-02$0$0$3.212750e+03$kg/h$5257$#EngIntakeAirMassFlowRate$16$16$1$2$1$0$5.000000e-02$0$0$3.212750e+03$kg/h$132$#  NSignals=3  StartBits=str2num('[double(0);double(32);double(16)]')  SignalSizes=str2num('[double(16),double(16),double(16)]')  ByteOrders=str2num('[int32(1);int32(1);int32(1)]')  DataTypes=str2num('[int32(2);int32(2);int32(2)]')  MultiplexTypes=str2num('[int32(1);int32(1);int32(1)]')  MultiplexValues=str2num('[double(0);double(0);double(0)]')  Factors=str2num('[double(5.000000e-02);double(5.000000e-02);double(5.000000e-02)]')  Offsets=str2num('[double(0);double(0);double(0)]')  Minimums=str2num('[double(0);double(0);double(0)]')  Maximums=str2num('[double(3.212750e+03);double(3.212750e+03);double(3.212750e+03)]')  Units=0  SPN=str2num('[double(2659);double(5257);double(132)]')  Comment=0  PGPriority=3  DestAddrID=Custom  DestAddrName=255  TransmitPeriodically=on  MessagePeriod=0  SampleTime=can_sample_time  ApplyMinMax=off
  J1939 Transmit4 : j1939protocollib/J1939 Transmit  Priority=-1  ConfigName=Config1  NodeName=Engine1  PGList=IMT1(65190)  PGName=IMT1  MsgLength=8  SignalInfo=EngTurbo1BoostPress$0$16$1$2$1$0$1.250000e-01$0$0$8.031875e+03$kPa$1127$#EngTurbo2BoostPress$16$16$1$2$1$0$1.250000e-01$0$0$8.031875e+03$kPa$1128$#EngTurbo3BoostPress$32$16$1$2$1$0$1.250000e-01$0$0$8.031875e+03$kPa$1129$#EngTurbo4BoostPress$48$16$1$2$1$0$1.250000e-01$0$0$8.031875e+03$kPa$1130$#  NSignals=4  StartBits=str2num('[double(0);double(16);double(32);double(48)]')  SignalSizes=str2num('[double(16),double(16),double(16),double(16)]')  ByteOrders=str2num('[int32(1);int32(1);int32(1);int32(1)]')  DataTypes=str2num('[int32(2);int32(2);int32(2);int32(2)]')  MultiplexTypes=str2num('[int32(1);int32(1);int32(1);int32(1)]')  MultiplexValues=str2num('[double(0);double(0);double(0);double(0)]')  Factors=str2num('[double(1.250000e-01);double(1.250000e-01);double(1.250000e-01);double(1.250000e-01)]')  Offsets=str2num('[double(0);double(0);double(0);double(0)]')  Minimums=str2num('[double(0);double(0);double(0);double(0)]')  Maximums=str2num('[double(8.031875e+03);double(8.031875e+03);double(8.031875e+03);double(8.031875e+03)]')  Units=0  SPN=str2num('[double(1127);double(1128);double(1129);double(1130)]')  Comment=0  PGPriority=6  DestAddrID=Custom  DestAddrName=255  TransmitPeriodically=on  MessagePeriod=0  SampleTime=can_sample_time  ApplyMinMax=off
  J1939 Transmit5 : j1939protocollib/J1939 Transmit  Priority=-1  ConfigName=Config1  NodeName=Engine1  PGList=ESSI(61473)  PGName=ESSI  MsgLength=8  SignalInfo=EngSpdSnsor1TimingPatternStatus$54$2$1$2$1$0$1$0$0$3$$4203$#EngSpdSnsor2TimingPatternStatus$52$2$1$2$1$0$1$0$0$3$$4204$#EngSpdSnsor3TimingPatternStatus$50$2$1$2$1$0$1$0$0$3$$4205$#EngSpeed1$0$16$1$2$1$0$5.000000e-01$0$0$3.212750e+04$rpm$4201$#EngSpeed2$16$16$1$2$1$0$5.000000e-01$0$0$3.212750e+04$rpm$723$#EngSpeed3$32$16$1$2$1$0$5.000000e-01$0$0$3.212750e+04$rpm$4202$#  NSignals=6  StartBits=str2num('[double(54);double(52);double(50);double(0);double(16);double(32)]')  SignalSizes=str2num('[double(2),double(2),double(2),double(16),double(16),double(16)]')  ByteOrders=str2num('[int32(1);int32(1);int32(1);int32(1);int32(1);int32(1)]')  DataTypes=str2num('[int32(2);int32(2);int32(2);int32(2);int32(2);int32(2)]')  MultiplexTypes=str2num('[int32(1);int32(1);int32(1);int32(1);int32(1);int32(1)]')  MultiplexValues=str2num('[double(0);double(0);double(0);double(0);double(0);double(0)]')  Factors=str2num('[double(1);double(1);double(1);double(5.000000e-01);double(5.000000e-01);double(5.000000e-01)]')  Offsets=str2num('[double(0);double(0);double(0);double(0);double(0);double(0)]')  Minimums=str2num('[double(0);double(0);double(0);double(0);double(0);double(0)]')  Maximums=str2num('[double(3);double(3);double(3);double(3.212750e+04);double(3.212750e+04);double(3.212750e+04)]')  Units=0  SPN=str2num('[double(4203);double(4204);double(4205);double(4201);double(723);double(4202)]')  Comment=0  PGPriority=6  DestAddrID=Custom  DestAddrName=255  TransmitPeriodically=on  MessagePeriod=0  SampleTime=can_sample_time  ApplyMinMax=off
  J1939 Transmit6 : j1939protocollib/J1939 Transmit  Priority=-1  ConfigName=Config1  NodeName=Engine1  PGList=ETC2(61445)  PGName=ETC2  MsgLength=8  SignalInfo=TransActualGearRatio$8$16$1$2$1$0$1.000000e-03$0$0$6.425500e+01$$526$#TransCurrentGear$24$8$1$2$1$0$1$-125$-125$125$$523$#TransCurrentRange$48$16$1$2$1$0$1$0$0$255$$163$#TransRqedRange$32$16$1$2$1$0$1$0$0$255$per$162$#TransSelectedGear$0$8$1$2$1$0$1$-125$-125$125$$524$#  NSignals=5  StartBits=str2num('[double(8);double(24);double(48);double(32);double(0)]')  SignalSizes=str2num('[double(16),double(8),double(16),double(16),double(8)]')  ByteOrders=str2num('[int32(1);int32(1);int32(1);int32(1);int32(1)]')  DataTypes=str2num('[int32(2);int32(2);int32(2);int32(2);int32(2)]')  MultiplexTypes=str2num('[int32(1);int32(1);int32(1);int32(1);int32(1)]')  MultiplexValues=str2num('[double(0);double(0);double(0);double(0);double(0)]')  Factors=str2num('[double(1.000000e-03);double(1);double(1);double(1);double(1)]')  Offsets=str2num('[double(0);double(-125);double(0);double(0);double(-125)]')  Minimums=str2num('[double(0);double(-125);double(0);double(0);double(-125)]')  Maximums=str2num('[double(6.425500e+01);double(125);double(255);double(255);double(125)]')  Units=0  SPN=str2num('[double(526);double(523);double(163);double(162);double(524)]')  Comment=0  PGPriority=6  DestAddrID=Custom  DestAddrName=255  TransmitPeriodically=on  MessagePeriod=0  SampleTime=can_sample_time  ApplyMinMax=off
  J1939 Transmit7 : j1939protocollib/J1939 Transmit  Priority=-1  ConfigName=Config1  NodeName=Engine1  PGList=CCVS(65265)  PGName=CCVS  MsgLength=8  SignalInfo=BrakeSwitch$28$2$1$2$1$0$1$0$0$3$$597$#ClutchSwitch$30$2$1$2$1$0$1$0$0$3$$598$#CruiseCtrlAccelerateSwitch$38$2$1$2$1$0$1$0$0$3$$602$#CruiseCtrlActive$24$2$1$2$1$0$1$0$0$3$$595$#CruiseCtrlCoastSwitch$34$2$1$2$1$0$1$0$0$3$$600$#CruiseCtrlEnableSwitch$26$2$1$2$1$0$1$0$0$3$$596$#CruiseCtrlPauseSwitch$4$2$1$2$1$0$1$0$0$3$$1633$#CruiseCtrlResumeSwitch$36$2$1$2$1$0$1$0$0$3$$601$#CruiseCtrlSetSpeed$40$8$1$2$1$0$1$0$0$250$km/h$86$#CruiseCtrlSetSwitch$32$2$1$2$1$0$1$0$0$3$$599$#CruiseCtrlStates$53$3$1$2$1$0$1$0$0$7$$527$#EngIdleDecrementSwitch$58$2$1$2$1$0$1$0$0$3$$967$#EngIdleIncrementSwitch$56$2$1$2$1$0$1$0$0$3$$968$#EngShutdownOverrideSwitch$62$2$1$2$1$0$1$0$0$3$$1237$#EngTestModeSwitch$60$2$1$2$1$0$1$0$0$3$$966$#PTOGovernorState$48$5$1$2$1$0$1$0$0$31$$976$#ParkBrakeReleaseInhibitRq$6$2$1$2$1$0$1$0$0$3$$3807$#ParkingBrakeSwitch$2$2$1$2$1$0$1$0$0$3$$70$#TwoSpeedAxleSwitch$0$2$1$2$1$0$1$0$0$3$$69$#WheelBasedVehicleSpeed$8$16$1$2$1$0$3.906250e-03$0$0$2.509960e+02$km/h$84$#  NSignals=20  StartBits=str2num('[double(28);double(30);double(38);double(24);double(34);double(26);double(4);double(36);double(40);double(32);double(53);double(58);double(56);double(62);double(60);double(48);double(6);double(2);double(0);double(8)]')  SignalSizes=str2num('[double(2),double(2),double(2),double(2),double(2),double(2),double(2),double(2),double(8),double(2),double(3),double(2),double(2),double(2),double(2),double(5),double(2),double(2),double(2),double(16)]')  ByteOrders=str2num('[int32(1);int32(1);int32(1);int32(1);int32(1);int32(1);int32(1);int32(1);int32(1);int32(1);int32(1);int32(1);int32(1);int32(1);int32(1);int32(1);int32(1);int32(1);int32(1);int32(1)]')  DataTypes=str2num('[int32(2);int32(2);int32(2);int32(2);int32(2);int32(2);int32(2);int32(2);int32(2);int32(2);int32(2);int32(2);int32(2);int32(2);int32(2);int32(2);int32(2);int32(2);int32(2);int32(2)]')  MultiplexTypes=str2num('[int32(1);int32(1);int32(1);int32(1);int32(1);int32(1);int32(1);int32(1);int32(1);int32(1);int32(1);int32(1);int32(1);int32(1);int32(1);int32(1);int32(1);int32(1);int32(1);int32(1)]')  MultiplexValues=str2num('[double(0);double(0);double(0);double(0);double(0);double(0);double(0);double(0);double(0);double(0);double(0);double(0);double(0);double(0);double(0);double(0);double(0);double(0);double(0);double(0)]')  Factors=str2num('[double(1);double(1);double(1);double(1);double(1);double(1);double(1);double(1);double(1);double(1);double(1);double(1);double(1);double(1);double(1);double(1);double(1);double(1);double(1);double(3.906250e-03)]')  Offsets=str2num('[double(0);double(0);double(0);double(0);double(0);double(0);double(0);double(0);double(0);double(0);double(0);double(0);double(0);double(0);double(0);double(0);double(0);double(0);double(0);double(0)]')  Minimums=str2num('[double(0);double(0);double(0);double(0);double(0);double(0);double(0);double(0);double(0);double(0);double(0);double(0);double(0);double(0);double(0);double(0);double(0);double(0);double(0);double(0)]')  Maximums=str2num('[double(3);double(3);double(3);double(3);double(3);double(3);double(3);double(3);double(250);double(3);double(7);double(3);double(3);double(3);double(3);double(31);double(3);double(3);double(3);double(2.509960e+02)]')  Units=0  SPN=str2num('[double(597);double(598);double(602);double(595);double(600);double(596);double(1633);double(601);double(86);double(599);double(527);double(967);double(968);double(1237);double(966);double(976);double(3807);double(70);double(69);double(84)]')  Comment=0  PGPriority=6  DestAddrID=Custom  DestAddrName=255  TransmitPeriodically=on  MessagePeriod=0  SampleTime=can_sample_time  ApplyMinMax=off
  Pulse Generator : DiscretePulseGenerator  PulseType=Time based  Period=can_sample_time*10  PulseWidth=10
  Rate Transition : RateTransition  OutPortSampleTime=control.Ts
  Scope : Scope
  Scope1 : Scope
  Scope2 : Scope
  Signal Generator : SignalGenerator  Commented=on  WaveForm=square  Amplitude=10  Frequency=0.01
  Signals3 : Scope  NumInputPorts=4
  Signals4 : Scope  NumInputPorts=4
  String Constant : StringConstant  String="\"D\""
  String Constant1 : StringConstant  String="\"4\""
  String to ASCII : StringToASCII
  String to ASCII1 : StringToASCII
  Terminator{,1..17} (18 alike) : Terminator
  To Workspace1 : ToWorkspace  VariableName=v_attack  SaveFormat=Timeseries  SampleTime=-1
  To Workspace2 : ToWorkspace  VariableName=v_chassis  SaveFormat=Timeseries  SampleTime=-1
  Velocity input : Scope
  Waveform Generator : simulink/Sources/Waveform Generator  Commented=on  OutMin=[]  OutMax=[]  OutDataTypeStr=double  SelectedSignal=1  BlockNames=MultiportSwitch_e3df3653d217406  SampleTime=0.1
  dummy 1 : Constant  Value=1996.85
  dummy 2 : Constant  Value=3
  dummy 3 : Constant  Value=6.463
  rx Vehicle Velocity : Outport
  rx Clutch Position : Outport  Port=2
  rx Inlet Manifold Pressure : Outport  Port=3
  rx trip distance : Outport  Port=4
  rx Compressor Air Mass Flow : Outport  Port=5
  rx Engine Speed : Outport  Port=6
  rx Current Gear : Outport  Port=7
  n_t : Outport  Port=8
  r_egr : Outport  Port=9
  lambda : Outport  Port=10
  k_slope : Outport  Port=11
  wires:
  clutch_pos/1 -> Data Type Conversion3/1
  "CAN Rx 65265 (Velocity, Clutch Pos)"/1(rx Vehicle Velocity) -> ?
  Data Type Conversion1/1 -> J1939 Transmit1/1
  Data Type Conversion2/1 -> J1939 Transmit1/2
  Vehicle Distance/1 -> Data Type Conversion1/1, Data Type Conversion2/1, Data Type Conversion5/1, Data Type Conversion4/1
  Data Type Conversion4/1 -> J1939 Transmit2/1
  Data Type Conversion5/1 -> J1939 Transmit2/2
  Inlet Manifold Pressure/1 -> J1939 Transmit4/3, J1939 Transmit4/4, J1939 Transmit4/2, J1939 Transmit4/1
  Compressor Air Mass Flow/1 -> J1939 Transmit3/3
  dummy 1/1 -> J1939 Transmit3/2, J1939 Transmit3/1
  Engine Speed/1 -> Scope/1, J1939 Transmit5/6, J1939 Transmit5/5, J1939 Transmit5/4
  dummy 2/1 -> J1939 Transmit5/2, J1939 Transmit5/1, J1939 Transmit5/3
  String Constant/1 -> String to ASCII/1
  String to ASCII/1 -> J1939 Transmit6/4
  String to ASCII1/1 -> J1939 Transmit6/3
  String Constant1/1 -> String to ASCII1/1
  dummy 3/1 -> J1939 Transmit6/1
  Current Gear/1 -> J1939 Transmit6/5, J1939 Transmit6/2
  "CAN Rx 65265 (Velocity, Clutch Pos)"/2(rx Clutch Pos) -> ?
  J1939 Receive2/2 -> rx trip distance/1
  J1939 Receive3/1 -> rx Inlet Manifold Pressure/1
  J1939 Receive4/3 -> rx Compressor Air Mass Flow/1
  J1939 Receive6/2 -> rx Current Gear/1
  J1939 Receive6/5 -> Terminator/1
  J1939 Receive6/4 -> Terminator1/1
  J1939 Receive6/3 -> Terminator2/1
  J1939 Receive6/1 -> Terminator3/1
  J1939 Receive5/6 -> Terminator4/1
  J1939 Receive5/5 -> Terminator5/1
  J1939 Receive5/3 -> Terminator6/1
  J1939 Receive5/2 -> Terminator7/1
  J1939 Receive5/1 -> Terminator8/1
  J1939 Receive4/2 -> Terminator9/1
  J1939 Receive4/1 -> Terminator10/1
  J1939 Receive3/4 -> Terminator11/1
  J1939 Receive3/3 -> Terminator12/1
  J1939 Receive3/2 -> Terminator13/1
  J1939 Receive1/2 -> Terminator14/1
  J1939 Receive1/1 -> Terminator15/1
  J1939 Receive2/1 -> Terminator16/1
  J1939 Receive7/20 -> Rate Transition/1
  J1939 Receive7/16 -> Signals3/1
  J1939 Receive7/9 -> Signals3/3
  J1939 Receive7/2 -> rx Clutch Position/1, Signals3/2
  Data Type Conversion3/1 -> J1939 Transmit7/2, Signals4/2
  Pulse Generator/1 -> Denial of Service/2, J1939 Transmit7/21, J1939 Transmit4/5, J1939 Transmit3/4, J1939 Transmit6/6, J1939 Transmit5/7, J1939 Transmit2/3, J1939 Transmit1/3, "CAN Tx 65265 (Velocity, Clutch Pos)"/3(trigger)  "Trigger"
  Data Type Conversion20/1 -> Signals4/4, J1939 Transmit7/20
  J1939 Receive5/4 -> Scope1/1, rx Engine Speed/1
  n_t_in/1 -> n_t/1
  r_egr_in/1 -> r_egr/1
  lambda_in/1 -> lambda/1
  k_slope_in/1 -> k_slope/1
  Dumy Inputs for CCVS Transmit block/18(Out18) -> Signals4/3
  Dumy Inputs for CCVS Transmit block/17(Out17) -> J1939 Transmit7/16, Signals4/1
  Dumy Inputs for CCVS Transmit block/1(Out1) -> J1939 Transmit7/1
  Dumy Inputs for CCVS Transmit block/2(Out2) -> J1939 Transmit7/3
  Dumy Inputs for CCVS Transmit block/3(Out3) -> J1939 Transmit7/4
  Dumy Inputs for CCVS Transmit block/4(Out4) -> J1939 Transmit7/5
  Dumy Inputs for CCVS Transmit block/5(Out5) -> J1939 Transmit7/6
  Dumy Inputs for CCVS Transmit block/6(Out6) -> J1939 Transmit7/7
  Dumy Inputs for CCVS Transmit block/7(Out7) -> J1939 Transmit7/8
  Dumy Inputs for CCVS Transmit block/8(Out8) -> J1939 Transmit7/10
  Dumy Inputs for CCVS Transmit block/9(Out9) -> J1939 Transmit7/11
  Dumy Inputs for CCVS Transmit block/10(Out10) -> J1939 Transmit7/12
  Dumy Inputs for CCVS Transmit block/11(Out11) -> J1939 Transmit7/13
  Dumy Inputs for CCVS Transmit block/12(Out12) -> J1939 Transmit7/14
  Dumy Inputs for CCVS Transmit block/13(Out13) -> J1939 Transmit7/15
  Dumy Inputs for CCVS Transmit block/14(Out14) -> J1939 Transmit7/17
  Dumy Inputs for CCVS Transmit block/15(Out15) -> J1939 Transmit7/18
  Dumy Inputs for CCVS Transmit block/16(Out16) -> J1939 Transmit7/19
  J1939 Receive7/1 -> Dummy Outputs/1(In1)
  J1939 Receive7/3 -> Dummy Outputs/2(In2)
  J1939 Receive7/4 -> Dummy Outputs/3(In3)
  J1939 Receive7/5 -> Dummy Outputs/4(In4)
  J1939 Receive7/6 -> Dummy Outputs/5(In5)
  J1939 Receive7/7 -> Dummy Outputs/6(In6)
  J1939 Receive7/8 -> Dummy Outputs/7(In7)
  J1939 Receive7/10 -> Dummy Outputs/8(In8)
  J1939 Receive7/11 -> Dummy Outputs/9(In9)
  J1939 Receive7/12 -> Dummy Outputs/10(In10)
  J1939 Receive7/13 -> Dummy Outputs/11(In11)
  J1939 Receive7/14 -> Dummy Outputs/12(In12)
  J1939 Receive7/15 -> Dummy Outputs/13(In13)
  J1939 Receive7/17 -> Dummy Outputs/14(In14)
  J1939 Receive7/18 -> Dummy Outputs/15(In15)
  J1939 Receive7/19 -> Dummy Outputs/16(In16)
  v_vehicle/1 -> To Workspace2/1, Attack Block/1(veloctiy)
  cruise_set_speed/1 -> Attack Block/2(Cruise_set_point), J1939 Transmit7/9
  Signal Generator/1 -> ?
  GAttack Block/1 -> ?
  Rate Transition/1 -> rx Vehicle Velocity/1, Signals3/4
  Constant2/1 -> Denial of Service/1
  J1939 Receive/1 -> Terminator17/1
  J1939 Receive/2 -> Scope2/1
  Attack Block/1(Out1) -> To Workspace1/1, Velocity input/1, Data Type Conversion20/1
